simulink model "Test"  (Simulink 4.00)
settings: Solver=ode45  StartTime=0.0  StopTime=1  RelTol=1e-3
values from neighbouring files (symbols this model uses):
  Pload = 200    [DP3.m]    (also in DP4.m; DP5.m)

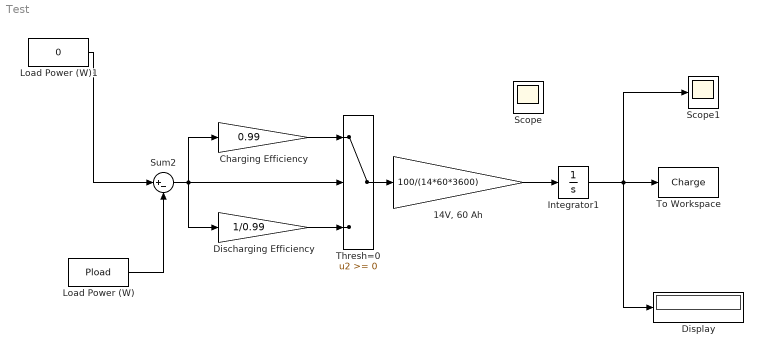
== system Test ==
  "14V, 60 Ah" : Gain  Gain=100/(14*60*3600)  Multiplication=Element-wise(K.*u)  SaturateOnIntegerOverflow=on
  Charging Efficiency : Gain  Gain=0.99  Multiplication=Element-wise(K.*u)  SaturateOnIntegerOverflow=on
  Discharging Efficiency : Gain  Gain=1/0.99  Multiplication=Element-wise(K.*u)  SaturateOnIntegerOverflow=on
  Display : Display
      settings: Format=short
  Integrator1 : Integrator  ExternalReset=none  InitialConditionSource=internal  InitialCondition=3  LimitOutput=off  UpperSaturationLimit=inf  LowerSaturationLimit=-inf  ShowSaturationPort=off  ShowStatePort=off  AbsoluteTolerance=auto
  Load Power (W) : Constant  Value=Pload
  Load Power (W)1 : Constant  Value=0
  Scope : Scope
      settings: TimeRange=auto  YMin=-5  YMax=5  SaveToWorkspace=off  SaveName=ScopeData  LimitDataPoints=on  MaxDataPoints=5000
  Scope1 : Scope
      settings: TimeRange=auto  YMin=-5  YMax=5  SaveToWorkspace=off  LimitDataPoints=on  MaxDataPoints=5000
  Sum2 : Sum  Inputs=|+-  SaturateOnIntegerOverflow=on
  Thresh=0 : Switch  Threshold=0
  To Workspace : ToWorkspace  VariableName=Charge  SampleTime=-1  SaveFormat=Array
  wires:
  Load Power (W)1/1 -> Sum2/1
  Load Power (W)/1 -> Sum2/2
  Charging Efficiency/1 -> Thresh=0/1
  Sum2/1 -> Charging Efficiency/1, Thresh=0/2, Discharging Efficiency/1
  Discharging Efficiency/1 -> Thresh=0/3
  "14V, 60 Ah"/1 -> Integrator1/1
  Integrator1/1 -> To Workspace/1, Scope1/1, Display/1
  Thresh=0/1 -> "14V, 60 Ah"/1
